simulink model "current_limiting_concept_plot"  (R2024b)
settings: Solver=VariableStepAuto  StartTime=0.0  StopTime=0.4  MaxStep=0.1e-3  RelTol=1e-3
InitFcn:
  | close all
  | clear all
StopFcn:
  | t = out.simout.time-0.05;
  | 
  | i_prelim = out.simout.signals.values(:,1);
  | i_limited = out.simout.signals.values(:,2);
  | 
  | plot_blanking = 1./(t>0.07) .* 1./(t<0.2);    % cheap trick to hide part of the curve
  | rms_limit_envelope = out.simout.signals.values(:,3) .* plot_blanking;
  | 
  | figure
  | plot(t, i_prelim, ...
  |     t, i_limited, ...
  |     t, rms_limit_envelope, '--r',...
  |     t, -rms_limit_envelope, '--r');
  | axis([-0.05, 0.25, -5, 5])
  | xlabel('time, seconds');
  | ylabel('current, pu');
  | legend('pre-limit', 'limited')
  | fig=gcf;
  | fig.Position(3:4)=[1000,400];
libraries: simulink x2
settings Model: Creator=HussamAlatrash  LastModifiedBy=HussamAlatrash

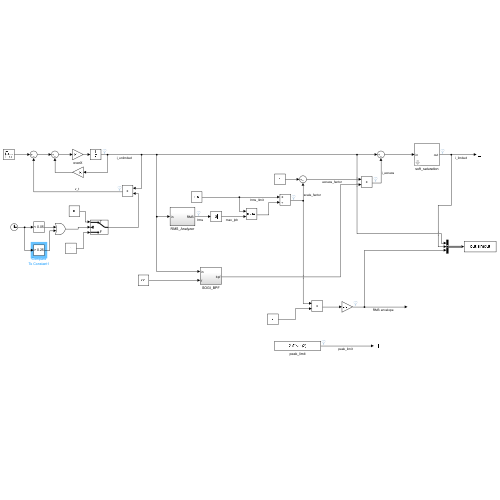
[thumbnail: Simulink's stored preview of the top-level diagram]
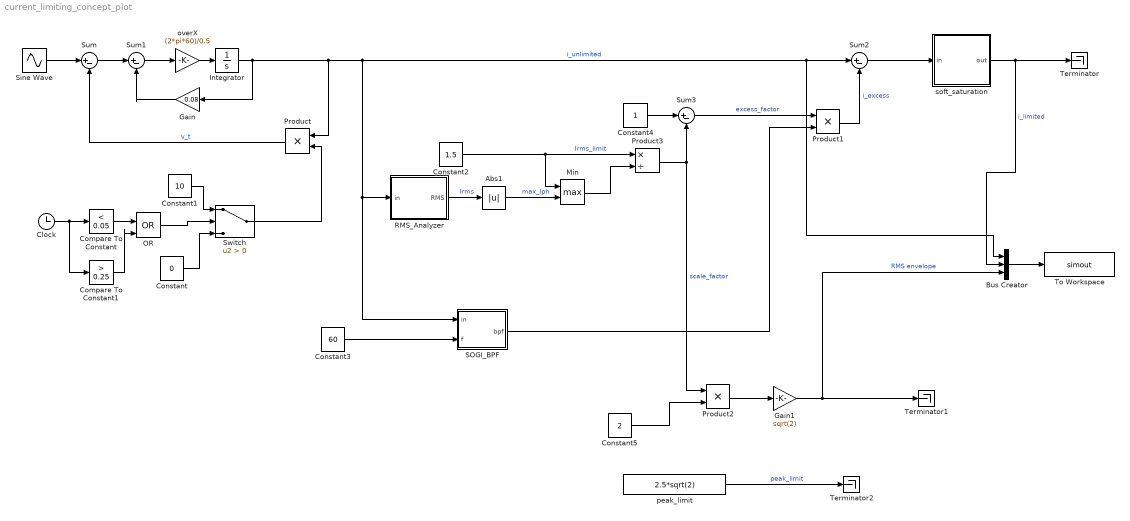
== system current_limiting_concept_plot ==
  Abs1 : Abs  SaturateOnIntegerOverflow=off
  Bus Creator : BusCreator  Inputs=3
  Clock : Clock
  Compare To Constant : simulink/Logic and Bit Operations/Compare To Constant  relop=<  const=0.05  OutDataTypeStr=boolean
  Compare To Constant1 : simulink/Logic and Bit Operations/Compare To Constant  relop=>  const=0.25  OutDataTypeStr=boolean
  Constant : Constant  Value=0
  Constant1 : Constant  Value=10
  Constant2 : Constant  Value=1.5
  Constant3 : Constant  Value=60
  Constant4 : Constant
  Constant5 : Constant  Value=2
  Gain : Gain  Gain=0.08
  Gain1 : Gain  Gain=sqrt(2)
  Integrator : Integrator
  Min : MinMax  Function=max  Inputs=2
  OR : Logic  Operator=OR  IconShape=distinctive  AllPortsSameDT=off  OutDataTypeStr=boolean
  Product : Product
  Product1 : Product
  Product2 : Product
  Product3 : Product  Inputs=*/
  RMS_Analyzer : Subsystem
  SOGI_BPF : Subsystem
  Sine Wave : Sin  Amplitude=1*sqrt(2)  Frequency=2*pi*60  SampleTime=0
  Sum{,1..3} (4 alike) : Sum  Inputs=|+-
  Switch : Switch  Criteria=u2 > Threshold  SaturateOnIntegerOverflow=off  InputSameDT=off
  Terminator : Terminator
  Terminator1 : Terminator
  Terminator2 : Terminator
  To Workspace : ToWorkspace  VariableName=simout  SaveFormat=Structure With Time  SampleTime=-1
  overX : Gain  Gain=(2*pi*60)/0.5
  peak_limit : Constant  Value=2.5*sqrt(2)
  soft_saturation : Subsystem  mask{soft_limit=1.8*sqrt(2), hard_limit=2.5*sqrt(2)}
      mask prompts: soft_limit "Soft limit"; hard_limit "Hard limit"
  wires:
  Sine Wave/1 -> Sum/1
  Sum/1 -> Sum1/1
  Integrator/1 -> SOGI_BPF/1(in), RMS_Analyzer/1(in), Bus Creator/1, Sum2/1, Product/1, Gain/1  "i_unlimited"
  Product/1 -> Sum/2  "v_t"
  Switch/1 -> Product/2
  overX/1 -> Integrator/1
  Sum1/1 -> overX/1
  Gain/1 -> Sum1/2
  Clock/1 -> Compare To Constant1/1, Compare To Constant/1
  OR/1 -> Switch/2
  Constant/1 -> Switch/3
  Constant1/1 -> Switch/1
  soft_saturation/1(out) -> Bus Creator/2, Terminator/1  "i_limited"
  RMS_Analyzer/1(RMS) -> Abs1/1  "Irms"
  SOGI_BPF/1(bpf) -> Product1/2
  Product1/1 -> Sum2/2  "i_excess"
  Sum2/1 -> soft_saturation/1(in)
  Constant3/1 -> SOGI_BPF/2(f)
  Min/1 -> Product3/2
  Constant4/1 -> Sum3/1
  Constant2/1 -> Product3/1, Min/1  "Irms_limit"
  Product3/1 -> Sum3/2, Product2/1  "scale_factor"
  Abs1/1 -> Min/2  "max_Iph"
  Sum3/1 -> Product1/1  "excess_factor"
  Product2/1 -> Gain1/1
  peak_limit/1 -> Terminator2/1  "peak_limit"
  Gain1/1 -> Bus Creator/3, Terminator1/1  "RMS envelope"
  Constant5/1 -> Product2/2
  Bus Creator/1 -> To Workspace/1
  Compare To Constant/1 -> OR/1
  Compare To Constant1/1 -> OR/2

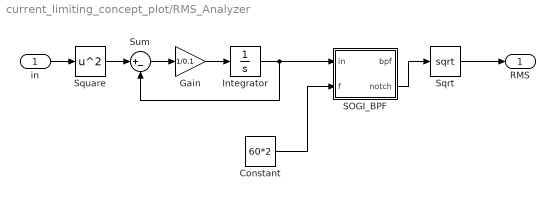
== system current_limiting_concept_plot/RMS_Analyzer ==
  in : Inport
  Constant : Constant  Value=60*2
  Gain : Gain  Gain=1/0.1
  Integrator : Integrator
  SOGI_BPF : Subsystem
  Sqrt : Sqrt
  Square : Math  Operator=square
  Sum : Sum  Inputs=|+-
  RMS : Outport
  wires:
  Square/1 -> Sum/1
  in/1 -> Square/1
  Gain/1 -> Integrator/1
  Sum/1 -> Gain/1
  Integrator/1 -> Sum/2, SOGI_BPF/1(in)
  Sqrt/1 -> RMS/1
  SOGI_BPF/2(notch) -> Sqrt/1
  Constant/1 -> SOGI_BPF/2(f)

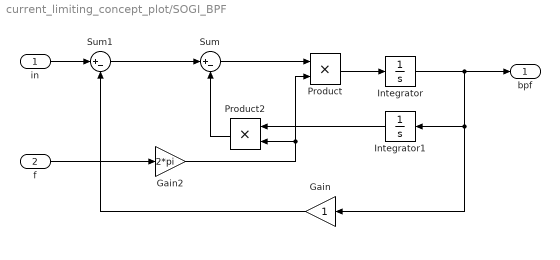
== system current_limiting_concept_plot/SOGI_BPF ==
  in : Inport
  f : Inport  Port=2
  Gain : Gain
  Gain2 : Gain  Gain=2*pi
  Integrator : Integrator
  Integrator1 : Integrator
  Product : Product
  Product2 : Product
  Sum : Sum  Inputs=|+-
  Sum1 : Sum  Inputs=|+-
  bpf : Outport
  wires:
  f/1 -> Gain2/1
  in/1 -> Sum1/1
  Product/1 -> Integrator/1
  Integrator1/1 -> Product2/1
  Gain/1 -> Sum1/2
  Sum1/1 -> Sum/1
  Integrator/1 -> Integrator1/1, Gain/1, bpf/1
  Gain2/1 -> Product2/2, Product/2
  Sum/1 -> Product/1
  Product2/1 -> Sum/2

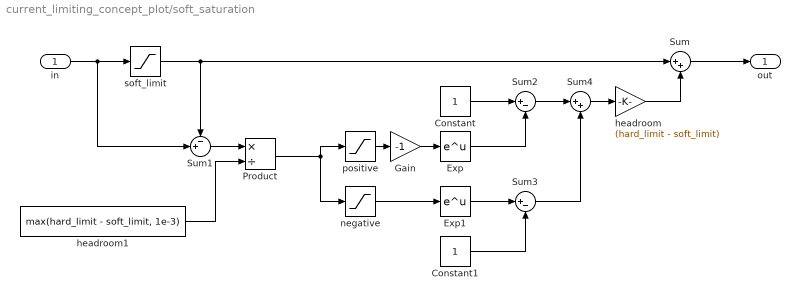
== system current_limiting_concept_plot/soft_saturation ==
  in : Inport
  Constant : Constant
  Constant1 : Constant
  Exp : Math
  Exp1 : Math
  Gain : Gain  Gain=-1
  Product : Product  Inputs=*/
  Sum : Sum  Inputs=|++
  Sum1 : Sum  Inputs=-+|
  Sum2 : Sum  Inputs=|+-
  Sum3 : Sum  Inputs=|+-
  Sum4 : Sum  Inputs=|++
  headroom : Gain  Gain=(hard_limit - soft_limit)
  headroom1 : Constant  Value=max(hard_limit - soft_limit, 1e-3)
  negative : Saturate  UpperLimit=0  LowerLimit=-inf
  positive : Saturate  UpperLimit=inf  LowerLimit=0
  soft_limit : Saturate  UpperLimit=soft_limit  LowerLimit=-soft_limit
  out : Outport
  wires:
  headroom1/1 -> Product/2
  Sum1/1 -> Product/1
  Sum2/1 -> Sum4/1
  Sum4/1 -> headroom/1
  Gain/1 -> Exp/1
  headroom/1 -> Sum/2
  Exp/1 -> Sum2/2
  positive/1 -> Gain/1
  in/1 -> soft_limit/1, Sum1/2
  Exp1/1 -> Sum3/1
  Sum/1 -> out/1
  soft_limit/1 -> Sum1/1, Sum/1
  Sum3/1 -> Sum4/2
  negative/1 -> Exp1/1
  Constant1/1 -> Sum3/2
  Product/1 -> positive/1, negative/1
  Constant/1 -> Sum2/1

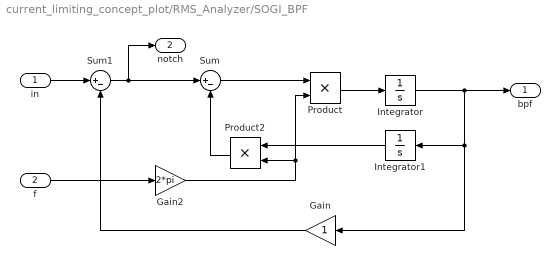
== system current_limiting_concept_plot/RMS_Analyzer/SOGI_BPF ==
  in : Inport
  f : Inport  Port=2
  Gain : Gain
  Gain2 : Gain  Gain=2*pi
  Integrator : Integrator
  Integrator1 : Integrator
  Product : Product
  Product2 : Product
  Sum : Sum  Inputs=|+-
  Sum1 : Sum  Inputs=|+-
  bpf : Outport
  notch : Outport  Port=2
  wires:
  f/1 -> Gain2/1
  in/1 -> Sum1/1
  Product/1 -> Integrator/1
  Integrator1/1 -> Product2/1
  Gain/1 -> Sum1/2
  Sum1/1 -> notch/1, Sum/1
  Integrator/1 -> Integrator1/1, Gain/1, bpf/1
  Gain2/1 -> Product2/2, Product/2
  Sum/1 -> Product/1
  Product2/1 -> Sum/2
